simulink model "p"  (Simulink 6.0)
settings: Solver=ode45  StartTime=0.0  StopTime=10.0  RelTol=1e-3
settings Model: LastModifiedBy=star

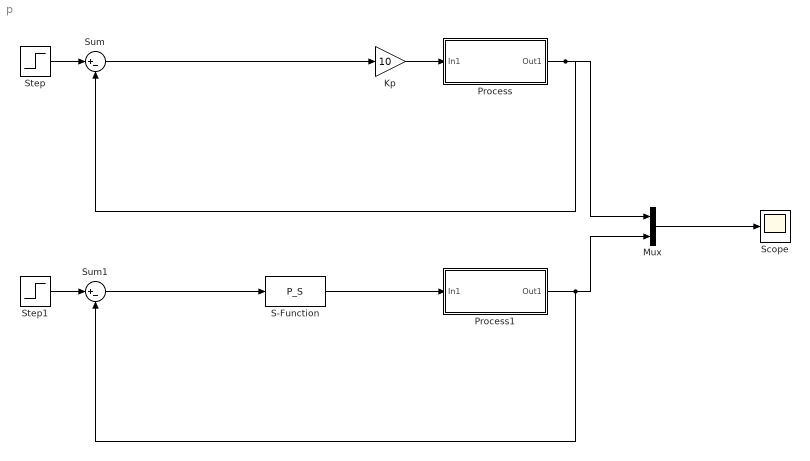
== system p ==
  Kp : Gain  Gain=10  SampleTime=0.01
  Mux : Mux  Inputs=2
  Process : Subsystem
  Process1 : Subsystem
  S-Function : S-Function  FunctionName=P_S  Parameters=0.01, 10
  Scope : Scope
  Step : Step  Time=0  SampleTime=0
  Step1 : Step  Time=0  SampleTime=0
  Sum : Sum  Inputs=|+-
  Sum1 : Sum  Inputs=|+-
  wires:
  Process/1(Out1) -> Sum/2, Mux/1
  Step/1 -> Sum/1
  Kp/1 -> Process/1(In1)
  Sum/1 -> Kp/1
  Process1/1(Out1) -> Sum1/2, Mux/2
  Step1/1 -> Sum1/1
  Mux/1 -> Scope/1
  Sum1/1 -> S-Function/1
  S-Function/1 -> Process1/1(In1)

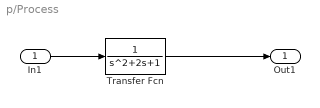
== system p/Process ==
  In1 : Inport  Port=1  LatchInput=off
  Transfer Fcn : TransferFcn
  Out1 : Outport
  wires:
  In1/1 -> Transfer Fcn/1
  Transfer Fcn/1 -> Out1/1

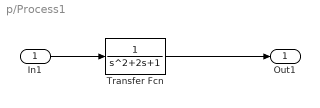
== system p/Process1 ==
  In1 : Inport  Port=1  LatchInput=off
  Transfer Fcn : TransferFcn
  Out1 : Outport
  wires:
  In1/1 -> Transfer Fcn/1
  Transfer Fcn/1 -> Out1/1
